simulink model "Octo_Model_15"  (Simulink 8.5)
settings: Solver=ode45  StartTime=0.0  StopTime=100  RelTol=1e-3
settings Model: Creator=utilisateur  LastModifiedBy=Majd
settings DataIOCC: SignalLoggingSaveFormat=Dataset
settings OptimizationCC: ExpressionDepthLimit=128
settings DebuggingCC: SolverPrmCheckMsg=warning  FcnCallInpInsideContextMsg=EnableAllAsError
settings GRTTargetCC: CombineOutputUpdateFcns=on  GRTInterface=off

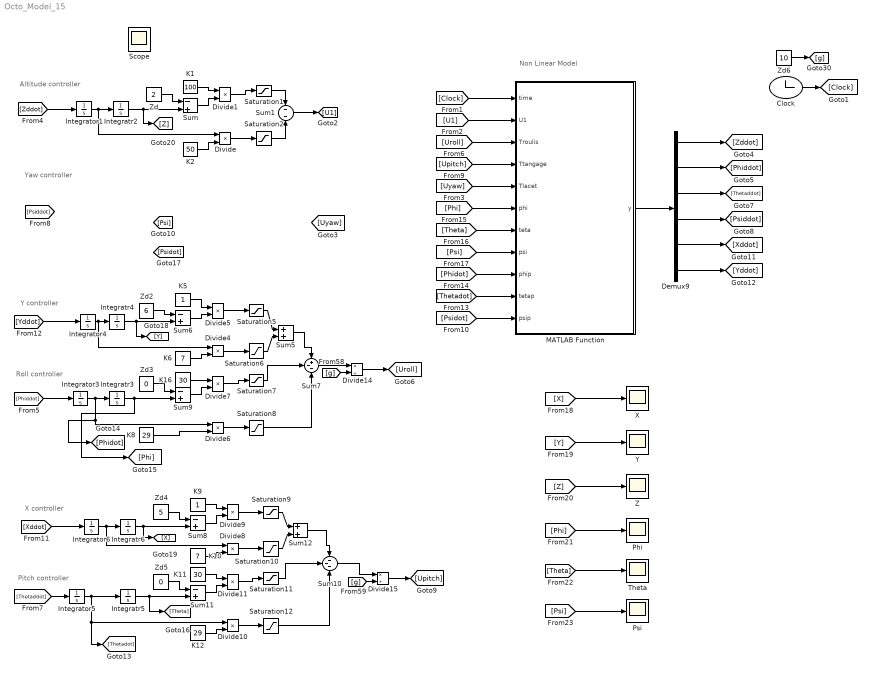
== system Octo_Model_15 ==
  note: Yaw controller
  note: Non Linear Model
  note: Pitch controller
  note: X controller
  note: Roll controller
  note: Y controller
  note: Altitude controller
  Clock : Clock
  Demux9 : Demux  Outputs=6
  Divide{,1,4..11} (10 alike) : Product  Inputs=**
  Divide14 : Product  Inputs=*/
  Divide15 : Product  Inputs=*/
  Integrator{1,3,5..6} (4 alike) : Integrator
  Integrator4 : Integrator  IgnoreLimit=on
  Integratr{2..3,5..6} (4 alike) : Integrator
  Integratr4 : Integrator  IgnoreLimit=on
  K1 : Constant  Value=100
  K10 : Constant  Value=7
  K11 : Constant  Value=30
  K12 : Constant  Value=29
  K16 : Constant  Value=30
  K2 : Constant  Value=50
  K5 : Constant
  K6 : Constant  Value=7
  K8 : Constant  Value=29
  K9 : Constant
  MATLAB Function : MATLAB Function  TreatAsAtomicUnit=on
      settings: PermitHierarchicalResolution=ParametersOnly
  Phi : Scope
      settings: TimeRange=auto  MaxDataPoints=5000  SaveToWorkspace=off  SaveName=ScopeData4  YMin=-0.10323  YMax=0.06505  SampleTime=-1
  Psi : Scope
      settings: TimeRange=auto  MaxDataPoints=5000  SaveToWorkspace=off  SaveName=ScopeData6  YMin=-0.00039  YMax=0.00004  SampleTime=-1
  Saturation{1..2,6..7} (4 alike) : Saturate  UpperLimit=20  LowerLimit=-20
  Saturation10 : Saturate  UpperLimit=8  LowerLimit=-8
  Saturation11 : Saturate  UpperLimit=15  LowerLimit=-15
  Saturation12 : Saturate  UpperLimit=30  LowerLimit=-30
  Saturation5 : Saturate  UpperLimit=15  LowerLimit=-15
  Saturation8 : Saturate  UpperLimit=30  LowerLimit=-30
  Saturation9 : Saturate  UpperLimit=6  LowerLimit=-6
  Sum{,6,8..9,11} (5 alike) : Sum  Inputs=-+
  Sum1 : Sum  Inputs=--
  Sum10 : Sum  Inputs=---
  Sum12 : Sum
  Sum5 : Sum
  Sum7 : Sum  Inputs=+--
  Theta : Scope
      settings: TimeRange=auto  MaxDataPoints=5000  SaveToWorkspace=off  SaveName=ScopeData5  YMin=-0.0542  YMax=0.08607  SampleTime=-1
  X : Scope
      settings: TimeRange=auto  MaxDataPoints=5000  SaveToWorkspace=off  YMin=-0.625  YMax=5.625  SampleTime=-1
  Y : Scope
      settings: TimeRange=auto  MaxDataPoints=5000  SaveToWorkspace=off  SaveName=ScopeData2  YMin=-0.75  YMax=6.75  SampleTime=-1
  Z : Scope
      settings: TimeRange=auto  MaxDataPoints=5000  SaveToWorkspace=off  SaveName=ScopeData3  YMin=-0.25  YMax=2.25  SampleTime=-1
  Zd : Constant  Value=2
  Zd2 : Constant  Value=6
  Zd3 : Constant  Value=0
  Zd4 : Constant  Value=5
  Zd5 : Constant  Value=0
  Zd6 : Constant  Value=10
  Scope : Scope
      settings: TimeRange=auto  MaxDataPoints=5000  SaveToWorkspace=off  SaveName=ScopeData  YMin=-0.6432  YMax=5.78876  SampleTime=-1
  wires:
  Zd/1 -> Sum/1
  K1/1 -> Divide1/1
  Sum/1 -> Divide1/2
  Divide1/1 -> Saturation1/1
  K2/1 -> Divide/2
  Divide/1 -> Saturation2/1
  Saturation2/1 -> Sum1/2
  Saturation1/1 -> Sum1/1
  Zd2/1 -> Sum6/1
  K5/1 -> Divide5/1
  Sum6/1 -> Divide5/2
  Divide5/1 -> Saturation5/1
  K6/1 -> Divide4/2
  Divide4/1 -> Saturation6/1
  Zd3/1 -> Sum9/1
  Sum9/1 -> Divide7/2
  Divide7/1 -> Saturation7/1
  Divide6/1 -> Saturation8/1
  Integrator1/1 -> Integratr2/1, Divide/1
  Integratr2/1 -> [Z], Sum/2
  Integrator3/1 -> [Phidot], Divide6/1, Integratr3/1
  Integrator4/1 -> Integratr4/1, Divide4/1
  Integratr4/1 -> [Y], Sum6/2
  [g] -> Divide14/2
  Zd4/1 -> Sum8/1
  K9/1 -> Divide9/1
  Sum8/1 -> Divide9/2
  Divide9/1 -> Saturation9/1
  K10/1 -> Divide8/2
  Divide8/1 -> Saturation10/1
  Zd5/1 -> Sum11/1
  K11/1 -> Divide11/1
  Sum11/1 -> Divide11/2
  Divide11/1 -> Saturation11/1
  K12/1 -> Divide10/2
  Divide10/1 -> Saturation12/1
  Integrator5/1 -> Divide10/1, [Thetadot], Integratr5/1
  Integratr5/1 -> [Theta], Sum11/2
  Integrator6/1 -> Integratr6/1, Divide8/1
  Integratr6/1 -> [X], Sum8/2
  [g] -> Divide15/2
  MATLAB Function/1(y) -> Demux9/1
  Sum7/1 -> Divide14/1
  Sum10/1 -> Divide15/1
  Integratr3/1 -> [Phi], Sum9/2
  Saturation8/1 -> Sum7/3
  Saturation7/1 -> Sum7/2
  Saturation6/1 -> Sum5/2
  Saturation5/1 -> Sum5/1
  Saturation12/1 -> Sum10/3
  Saturation11/1 -> Sum10/2
  Saturation9/1 -> Sum12/1
  Saturation10/1 -> Sum12/2
  K8/1 -> Divide6/2
  K16/1 -> Divide7/1
  Sum5/1 -> Sum7/1
  Sum12/1 -> Sum10/1
  Clock/1 -> [Clock]
  Zd6/1 -> [g]
  [Clock] -> MATLAB Function/1(time)
  Sum1/1 -> [U1]
  [U1] -> MATLAB Function/2(U1)
  [Uyaw] -> MATLAB Function/5(Tlacet)
  Demux9/1 -> [Zddot]
  [Zddot] -> Integrator1/1
  [Phiddot] -> Integrator3/1
  Demux9/2 -> [Phiddot]
  Divide14/1 -> [Uroll]
  [Uroll] -> MATLAB Function/3(Troulis)
  [Thetaddot] -> Integrator5/1
  Demux9/3 -> [Thetaddot]
  Demux9/4 -> [Psiddot]
  [Upitch] -> MATLAB Function/4(Ttangage)
  Divide15/1 -> [Upitch]
  [Psidot] -> MATLAB Function/11(psip)
  [Xddot] -> Integrator6/1
  Demux9/5 -> [Xddot]
  Demux9/6 -> [Yddot]
  [Yddot] -> Integrator4/1
  [Thetadot] -> MATLAB Function/10(tetap)
  [Phidot] -> MATLAB Function/9(phip)
  [Phi] -> MATLAB Function/6(phi)
  [Theta] -> MATLAB Function/7(teta)
  [Psi] -> MATLAB Function/8(psi)
  [X] -> X/1
  [Y] -> Y/1
  [Z] -> Z/1
  [Phi] -> Phi/1
  [Theta] -> Theta/1
  [Psi] -> Psi/1

== matlab function MATLAB Function ==
  data: time input double; U1 input double; Troulis input double; Ttangage input double; Tlacet input double; y output double; phi input double; teta input double; psi input double; phip input double; tetap input double; psip input double
% % Master Robotique et Systèmes Intelligents
% % RSI07-Diagnostic et Tolérance aux fautes des systèmes dynamiques
% % Décembre 2017

% *****************************************************************************************************************
% % Coaxial Octorotor UAV
% % Parameters of the Modulo-X octorotor at Heudiasyc Laboratory, UTC
% % Non linear Model, Altitude, Attitude and Position Control using PD with saturations


function y   = Octorotor_UAV(time,U1,Troulis,Ttangage,Tlacet,phi,teta,psi,phip,tetap,psip)

%****************************************************************************************************************************
% Octorotor Parameters
Jx=0.0255;  % Octorotor moment of inertia around X axis
Jy=0.0255;  % Octorotor moment of inertia around Y axis
Jz=0.0388;  % Octorotor moment of inertia around Z axis
Kf=3.5*10^-5; % Thrust factor
Kt=3*10^-7; % Reaction Torque coefficient
L=0.23; % length of the arm
m=1.6; % mass of the octorotor



U=(U1+10)*m/(cos(phi)*cos(teta));

%**************************************************************************
% % Motors Speeds

 W1=sqrt(max(0,(1/8)*(U/(Kf)-(Troulis)/(L*Kf)-Ttangage/(L*Kf)-Tlacet/(Kt))));
 W2=sqrt(max(0,(1/8)*(U/(Kf)-(Troulis)/(L*Kf)-Ttangage/(L*Kf)+Tlacet/(Kt))));
 W3=sqrt(max(0,(1/8)*(U/(Kf)-(Troulis)/(L*Kf)+Ttangage/(L*Kf)+Tlacet/(Kt))));
 W4=sqrt(max(0,(1/8)*(U/(Kf)-(Troulis)/(L*Kf)+Ttangage/(L*Kf)-Tlacet/(Kt))));
 W5=sqrt(max(0,(1/8)*(U/(Kf)+(Troulis)/(L*Kf)+Ttangage/(L*Kf)-Tlacet/(Kt))));
 W6=sqrt(max(0,(1/8)*(U/(Kf)+(Troulis)/(L*Kf)+Ttangage/(L*Kf)+Tlacet/(Kt))));
 W7=sqrt(max(0,(1/8)*(U/(Kf)+(Troulis)/(L*Kf)-Ttangage/(L*Kf)+Tlacet/(Kt))));
 W8=sqrt(max(0,(1/8)*(U/(Kf)+(Troulis)/(L*Kf)-Ttangage/(L*Kf)-Tlacet/(Kt))));
 

%**************************************************************************

% % Individual Thrusts and Torques

Z1=Kf*W1^2;T1=Kt*W1^2;
Z2=Kf*W2^2;T2=Kt*W2^2;
Z3=Kf*W3^2;T3=Kt*W3^2;
Z4=Kf*W4^2;T4=Kt*W4^2;
Z5=Kf*W5^2;T5=Kt*W5^2;
Z6=Kf*W6^2;T6=Kt*W6^2;
Z7=Kf*W7^2;T7=Kt*W7^2;
Z8=Kf*W8^2;T8=Kt*W8^2;
 
%*************************************************************************
% %Thrusts of coaxial motors
Z12=(Z1+Z2);
Z34=(Z3+Z4);
Z56=(Z5+Z6);
Z78=(Z7+Z8);
%*************************************************************************
% % Total Thrust
U_calcule=Z12+Z34+Z56+Z78;
%*************************************************************************
% % Roll, pitch and yaw moments
Troulis_calcule=((Z56+Z78)-(Z12+Z34))*L*sqrt(2)/2;
Ttangage_calcule=((Z34+Z56)-(Z12+Z78))*L*sqrt(2)/2;
Tlacet_calcule=(T2+T6+T3+T7)-(T1+T5+T4+T8);

%*************************************************************************
% % Non Linear Model of the octorotor UAV
fx=(cos(phi)*sin(teta)*cos(psi)+sin(phi)*sin(psi))*U_calcule/m;%(xpp)
fy= %(ypp)
fz= %(zpp)
fphi= %(phipp)
fteta= %(thetapp)
fpsi= %(psipp)
                                                                                                         
y=[fz,fphi,fteta,fpsi,fx,fy];
